simulink model "linear_seesaw_matlabsimulink_29_04_2024"  (R2023b)
settings: Solver=VariableStepAuto  StartTime=0.0  StopTime=3  FixedStep=3  RelTol=1e-3
values from neighbouring files (symbols this model uses):
  A = [0,mf*g*h/Jconst,0,-mf*g/Jconst; 1,0,0,0; 0,-g,0,0; 0,0,1,0]    [linear_seesaw_matlabsimulink_29_04_2024_inizalise.m]
  B = [1/Jconst;0;0;0]    [linear_seesaw_matlabsimulink_29_04_2024_inizalise.m]
  g = 9.81    [linear_seesaw_matlabsimulink_29_04_2024_inizalise.m]
  h = 0.1    [linear_seesaw_matlabsimulink_29_04_2024_inizalise.m]
  Jconst = mf*h^2+Jb    (= 0.501)    [linear_seesaw_matlabsimulink_29_04_2024_inizalise.m]
  mf = 0.1    [linear_seesaw_matlabsimulink_29_04_2024_inizalise.m]
settings Model: Creator=dmplab  LastModifiedBy=Krish
settings DebuggingCC: UnconnectedInputMsg=warning  UnconnectedOutputMsg=warning  UnconnectedLineMsg=warning
settings ModelReferenceCC: EnableRefExpFcnMdlSchedulingChecks=on
settings RTWCC: DLArmComputeVersion=19.05

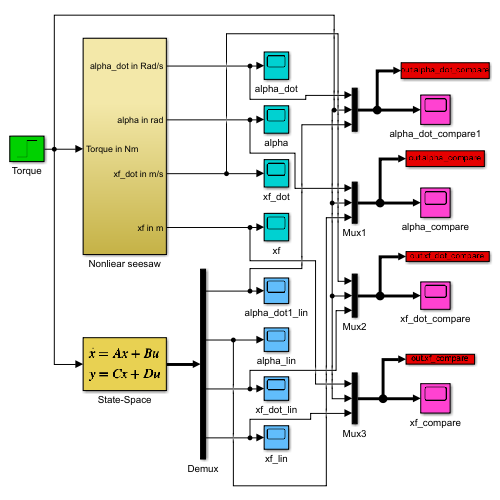
[thumbnail: Simulink's stored preview of the top-level diagram]
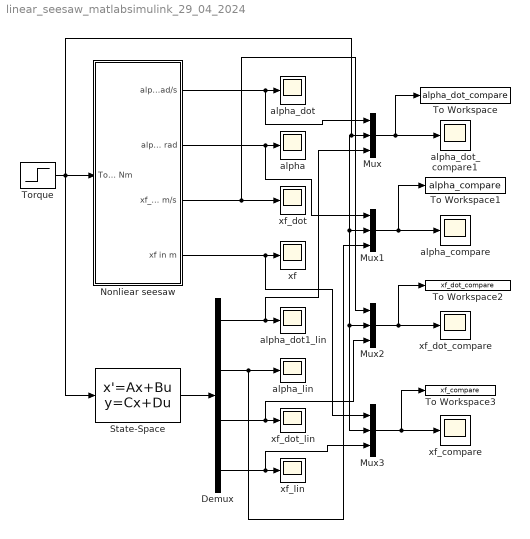
== system linear_seesaw_matlabsimulink_29_04_2024 ==
  Demux : Demux
  Mux{,1..3} (4 alike) : Mux  Inputs=3
  Nonliear seesaw : Subsystem
  State-Space : StateSpace  A=A  B=B  C=eye(4)  D=[0;0;0;0]  InitialCondition=0
  To Workspace : ToWorkspace  VariableName=alpha_dot_compare  SaveFormat=Timeseries  SampleTime=-1
  To Workspace1 : ToWorkspace  VariableName=alpha_compare  SaveFormat=Timeseries  SampleTime=-1
  To Workspace2 : ToWorkspace  VariableName=xf_dot_compare  SaveFormat=Timeseries  SampleTime=-1
  To Workspace3 : ToWorkspace  VariableName=xf_compare  SaveFormat=Timeseries  SampleTime=-1
  Torque : Step  SampleTime=0
  alpha : Scope
  alpha_compare : Scope
  alpha_dot : Scope
  alpha_dot1_lin : Scope
  alpha_dot_compare1 : Scope
  alpha_lin : Scope
  xf : Scope
  xf_compare : Scope
  xf_dot : Scope
  xf_dot_compare : Scope
  xf_dot_lin : Scope
  xf_lin : Scope
  wires:
  Torque/1 -> State-Space/1, Nonliear seesaw/1(Torque in Nm), Mux2/2, Mux3/2, Mux1/2, Mux/2
  Nonliear seesaw/2(alpha in rad) -> Mux1/1, alpha/1
  Nonliear seesaw/3(xf_dot in m/s) -> xf_dot/1, Mux2/1
  Nonliear seesaw/4(xf in m) -> Mux3/1, xf/1
  State-Space/1 -> Demux/1
  Demux/4 -> Mux3/3, xf_lin/1
  Demux/3 -> Mux2/3, xf_dot_lin/1
  Demux/2 -> alpha_lin/1, Mux1/3
  Demux/1 -> Mux/3, alpha_dot1_lin/1
  Nonliear seesaw/1(alpha_dot in Rad/s) -> Mux/1, alpha_dot/1
  Mux1/1 -> To Workspace1/1, alpha_compare/1
  Mux2/1 -> To Workspace2/1, xf_dot_compare/1
  Mux3/1 -> xf_compare/1, To Workspace3/1
  Mux/1 -> To Workspace/1, alpha_dot_compare1/1

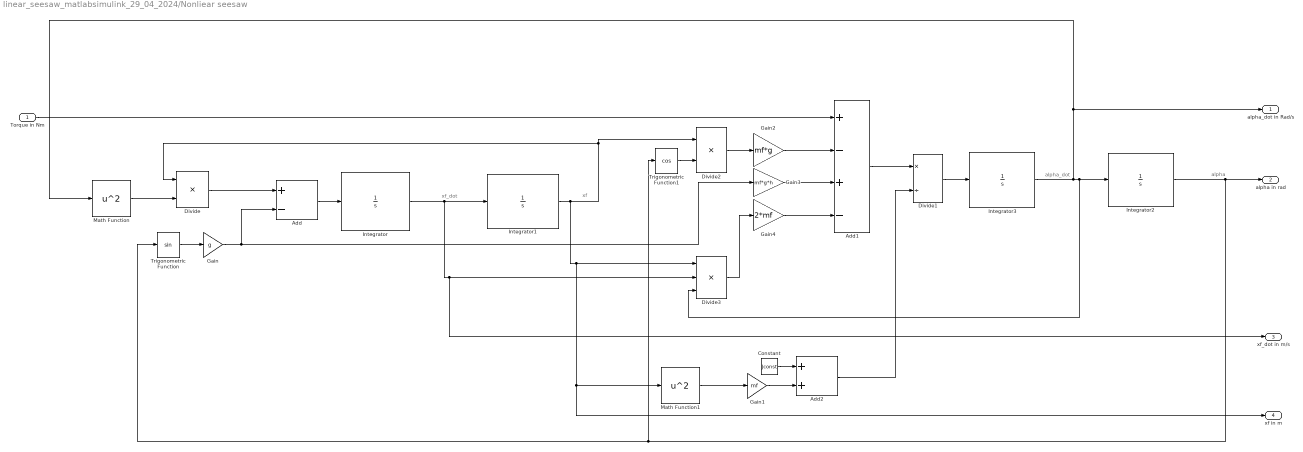
== system linear_seesaw_matlabsimulink_29_04_2024/Nonliear seesaw ==
  note: alpha_dot
  note: xf_dot
  note: xf
  note: alpha
  Torque in Nm : Inport
  Add : Sum  Inputs=+-
  Add1 : Sum  Inputs=+-+-
  Add2 : Sum
  Constant : Constant  Value=Jconst
  Divide : Product  Inputs=**
  Divide1 : Product  Inputs=*/
  Divide2 : Product  Inputs=**
  Divide3 : Product  Inputs=***
  Gain : Gain  Gain=g
  Gain1 : Gain  Gain=mf
  Gain2 : Gain  Gain=mf*g
  Gain3 : Gain  Gain=mf*g*h
  Gain4 : Gain  Gain=2*mf
  Integrator{,1..3} (4 alike) : Integrator
  Math Function : Math  Operator=square
  Math Function1 : Math  Operator=square
  Trigonometric Function : Trigonometry
  Trigonometric Function1 : Trigonometry  Operator=cos
  alpha_dot in Rad/s : Outport
  alpha in rad : Outport  Port=2
  xf_dot in m/s : Outport  Port=3
  xf in m : Outport  Port=4
  wires:
  Gain/1 -> Gain3/1, Add/2
  Integrator2/1 -> Trigonometric Function1/1, Trigonometric Function/1, alpha in rad/1
  Integrator/1 -> xf_dot in m/s/1, Divide3/2, Integrator1/1
  Integrator3/1 -> Integrator2/1, Divide3/3, alpha_dot in Rad/s/1, Math Function/1
  Divide/1 -> Add/1
  Integrator1/1 -> xf in m/1, Math Function1/1, Divide3/1, Divide/1, Divide2/1
  Constant/1 -> Add2/1
  Divide3/1 -> Gain4/1
  Gain2/1 -> Add1/2
  Math Function/1 -> Divide/2
  Add/1 -> Integrator/1
  Gain4/1 -> Add1/4
  Gain1/1 -> Add2/2
  Trigonometric Function/1 -> Gain/1
  Math Function1/1 -> Gain1/1
  Add1/1 -> Divide1/1
  Gain3/1 -> Add1/3
  Divide1/1 -> Integrator3/1
  Add2/1 -> Divide1/2
  Divide2/1 -> Gain2/1
  Trigonometric Function1/1 -> Divide2/2
  Torque in Nm/1 -> Add1/1
